simulink model "e5_3blocks_nn"  (R2020a)
settings: Solver=VariableStepAuto  StartTime=0.0  StopTime=10.0  RelTol=1e-3
undefined symbols (not defined in the file or in its folder): Quad
libraries: neural x123
(part 3 of 6)

== system e5_3blocks_nn/NN/Layer 2/Delays 1 ==
  "p{2}" : Inport  PortDimensions=50
      mask Display: e = 0.06;c1 = [120 230 180]/255;c2 = ([120 230 180]+0)/(256+128);c3 = ([120 230 180]+128)/(256+128);patch([0 1 1 0],[0 0 1 1],c1);patch([0 1 1 1-e 1-e 0+e],[0 0 1 1-e 0+e 0+e],c2);patch([0 0 1 1-e 0+e 0+e],[0 1 1 1-e 1-e 0+e],c3);plot([0 1 1 0 0],[0 0 1 1 0]);
  mux : Mux  Inputs=1
      mask Display: e = 0.06;c1 = [120 150 230]/255;c2 = ([120 150 230]+0)/383;c3 = ([120 150 230]+128)/383;patch([0 1 1 0],[0 0 1 1],c1);patch([0 1 1 1-e 1-e 0+e],[0 0 1 1-e 0+e 0+e],c2);patch([0 0 1 1-e 0+e 0+e],[0 1 1 1-e 1-e 0+e],c3);plot([0 1 1 0 0],[0 0 1 1 0]);disp('Mux')
  "pd{2,1}" : Outport
      mask Display: e = 0.06;c1 = [120 230 180]/255;c2 = ([120 230 180]+0)/(256+128);c3 = ([120 230 180]+128)/(256+128);patch([0 1 1 0],[0 0 1 1],c1);patch([0 1 1 1-e 1-e 0+e],[0 0 1 1-e 0+e 0+e],c2);patch([0 0 1 1-e 0+e 0+e],[0 1 1 1-e 1-e 0+e],c3);plot([0 1 1 0 0],[0 0 1 1 0]);
  wires:
  "p{2}"/1 -> mux/1
  mux/1 -> "pd{2,1}"/1

== system e5_3blocks_nn/NN/Layer 2/LW{2,1} ==
  "ad{2,1}" : Inport  PortDimensions=50
      mask Display: e = 0.06;c1 = [120 230 180]/255;c2 = ([120 230 180]+0)/(256+128);c3 = ([120 230 180]+128)/(256+128);patch([0 1 1 0],[0 0 1 1],c1);patch([0 1 1 1-e 1-e 0+e],[0 0 1 1-e 0+e 0+e],c2);patch([0 0 1 1-e 0+e 0+e],[0 1 1 1-e 1-e 0+e],c3);plot([0 1 1 0 0],[0 0 1 1 0]);
  "IW{2,1}(1,:)'" : Constant  Value=[0.06238826944898899495850486118797562085092067718505859375;-0.0662561883727814660005606128834187984466552734375;0.140596693924744442494301210899720899760723114013671875;0.3008382961340732020261157231288962066173553466796875;0.329270133314576940453122233520844019949436187744140625;-0.08899910732660483436706755355771747417747974395751953125;0.11667890650152978881948229172849096357822418212890625;-0.1929670553806901167614995529220323078334331512451171875;0.2111795311514239326111663785923155955970287322998046875;0.2287193471798081301216143401688896119594573974609375;-0.29845320395423546866453534676111303269863128662109375;-0.1754752706825663810530357977768289856612682342529296875;-0.234519474313424625133706058477400802075862884521484375;0.01548211534042116983844739053211014834232628345489501953125;-0.1728192200925544319556337313770200125873088836669921875;0.203750612111709583640362097867182455956935882568359375;-0.03263481715507744740367712665829458273947238922119140625;-0.0835109388646079475737593611484044231474399566650390625;-0.173454103671987935886278364705503918230533599853515625;-0.25354274639018326009676229659817181527614593505859375;0.05956454210532587112414404373339493758976459503173828125;-0.12377788023767373470906960619686287827789783477783203125;-0.048979806865181163555433840883779339492321014404296875;-0.0684319290588069339964505388707038946449756622314453125;0.2344023881326581515427420754349441267549991607666015625;0.0686577095032668005547549228140269406139850616455078125;0.0705147028712725665311467082574381493031978607177734375;0.311049450843584984749412569726700894534587860107421875;0.183230131462504053363460343462065793573856353759765625;0.081252526365822586029707963461987674236297607421875;-0.20765571332480303734513427116326056420803070068359375;0.02676877785194743675223350010128342546522617340087890625;0.30055041682881888931433422840200364589691162109375;0.09562847935589045833548738073659478686749935150146484375;0.1668647100894824486516654360457323491573333740234375;-0.0961144552936583351776533845622907392680644989013671875;-0.0312302350081472245013625155252157128416001796722412109375;-0.35432114836700978610650736300158314406871795654296875;0.1700429182737286104565299638124997727572917938232421875;-0.1468128720628165684303212401573546230792999267578125;0.32478039488932564093914834302267991006374359130859375;-0.2290287491159137822638314219148014672100543975830078125;-0.08672457421688405110327124702962464652955532073974609375;0.0266731992851400624700008989975685835815966129302978515625;0.1662091278922168957610239203859237022697925567626953125;0.2276717647203591876614581224202993325889110565185546875;0.199822119171683965088703871515463106334209442138671875;0.1305782909366972333042866694086114875972270965576171875;-0.0745158904154400725250440018498920835554599761962890625;-0.11266355005217280893514697481805342249572277069091796875]
      mask Display: e = 0.06;c1 = [120 150 230]/255;c2 = ([120 150 230]+0)/383;c3 = ([120 150 230]+128)/383;patch([0 1 1 0],[0 0 1 1],c1);patch([0 1 1 1-e 1-e 0+e],[0 0 1 1-e 0+e 0+e],c2);patch([0 0 1 1-e 0+e 0+e],[0 1 1 1-e 1-e 0+e],c3);plot([0 1 1 0 0],[0 0 1 1 0]);disp('weights');
  "IW{2,1}(2,:)'" : Constant  Value=[0.053859911191078267689302805365514359436929225921630859375;0.1116533205692238350792422352242283523082733154296875;-0.4240343441799243606737945810891687870025634765625;0.1368953708668934343695156030662474222481250762939453125;-0.0943260353503585780021722939636674709618091583251953125;0.171733416516677672714052960145636461675167083740234375;0.262014754263373450537955022809910587966442108154296875;0.04316320852678133535018645261516212485730648040771484375;-0.094505581266535354512114963654312305152416229248046875;0.1799789979013576568522836396368802525103092193603515625;-0.15630297243227875281235128568368963897228240966796875;0.12384955587173805680034632814567885361611843109130859375;0.1190447085715764241609093687657150439918041229248046875;0.263289083945134116948594282803242094814777374267578125;-0.1125910082716607141239961720202700234949588775634765625;-0.03594825728761497085628207059926353394985198974609375;-0.09538179906421283271722444396800710819661617279052734375;0.03382504542857060758631604358015465550124645233154296875;-0.09516068664822209532960783917587832547724246978759765625;-0.2472115131330177850710327902561402879655361175537109375;0.2200282479288944159634411334991455078125;-0.27077531053553050011117875328636728227138519287109375;0.11230775374953057277327417295964551158249378204345703125;0.10448450591650038088431529104127548635005950927734375;0.209030737108533870571847046448965556919574737548828125;-0.03888027185597515977821814203707617707550525665283203125;-0.2230029398786366190421404098742641508579254150390625;-0.2113154090177686850182681155274622142314910888671875;0.2253159625747749306157174942200072109699249267578125;-0.0759738296823943837221548847082885913550853729248046875;0.0232977391038076131479783725808374583721160888671875;0.0495270194348351455726486847197520546615123748779296875;-0.148411826106503053068763620103709399700164794921875;0.361210691757326285422635692157200537621974945068359375;-0.255217278371725975194550528613035567104816436767578125;-0.1139007461432639811693690035099280066788196563720703125;-0.131820962715450018531981868363800458610057830810546875;0.03699478200002949412894537317697540856897830963134765625;0.371812042058923708509610150940716266632080078125;0.238123332367356888017440041949157603085041046142578125;0.1813876888061571601706845058288308791816234588623046875;-0.04579007505833264379813130062757409177720546722412109375;-0.0142746944588547051979698920831651776097714900970458984375;-0.0505190325210966018065761318212025798857212066650390625;0.1416573248566437015494301476792315952479839324951171875;0.1885353697001486417139659579333965666592121124267578125;0.449669560775642296324150493092020042240619659423828125;0.07124427017188149358073445682748570106923580169677734375;0.0272623856827981791983717130278819240629673004150390625;-0.1683749712734463610530610822024755179882049560546875]
      mask Display: e = 0.06;c1 = [120 150 230]/255;c2 = ([120 150 230]+0)/383;c3 = ([120 150 230]+128)/383;patch([0 1 1 0],[0 0 1 1],c1);patch([0 1 1 1-e 1-e 0+e],[0 0 1 1-e 0+e 0+e],c2);patch([0 0 1 1-e 0+e 0+e],[0 1 1 1-e 1-e 0+e],c3);plot([0 1 1 0 0],[0 0 1 1 0]);disp('weights');
  Mux : Mux  Inputs=2
      mask Display: e = 0.06;c1 = [120 150 230]/255;c2 = ([120 150 230]+0)/383;c3 = ([120 150 230]+128)/383;patch([0 1 1 0],[0 0 1 1],c1);patch([0 1 1 1-e 1-e 0+e],[0 0 1 1-e 0+e 0+e],c2);patch([0 0 1 1-e 0+e 0+e],[0 1 1 1-e 1-e 0+e],c3);plot([0 1 1 0 0],[0 0 1 1 0]);disp('Mux');
  dotprod1 : neural/Weight Functions/dotprod
  dotprod2 : neural/Weight Functions/dotprod
  "lz{2,1}" : Outport
      mask Display: e = 0.06;c1 = [120 230 180]/255;c2 = ([120 230 180]+0)/(256+128);c3 = ([120 230 180]+128)/(256+128);patch([0 1 1 0],[0 0 1 1],c1);patch([0 1 1 1-e 1-e 0+e],[0 0 1 1-e 0+e 0+e],c2);patch([0 0 1 1-e 0+e 0+e],[0 1 1 1-e 1-e 0+e],c3);plot([0 1 1 0 0],[0 0 1 1 0]);
  wires:
  "IW{2,1}(1,:)'"/1 -> dotprod1/1
  "ad{2,1}"/1 -> dotprod1/2, dotprod2/2
  dotprod1/1 -> Mux/1
  "IW{2,1}(2,:)'"/1 -> dotprod2/1
  dotprod2/1 -> Mux/2
  Mux/1 -> "lz{2,1}"/1

== system e5_3blocks_nn/NN_online/Layer 1/Delays 1 ==
  "p{1}" : Inport  PortDimensions=20
      mask Display: e = 0.06;c1 = [120 230 180]/255;c2 = ([120 230 180]+0)/(256+128);c3 = ([120 230 180]+128)/(256+128);patch([0 1 1 0],[0 0 1 1],c1);patch([0 1 1 1-e 1-e 0+e],[0 0 1 1-e 0+e 0+e],c2);patch([0 0 1 1-e 0+e 0+e],[0 1 1 1-e 1-e 0+e],c3);plot([0 1 1 0 0],[0 0 1 1 0]);
  mux : Mux  Inputs=1
      mask Display: e = 0.06;c1 = [120 150 230]/255;c2 = ([120 150 230]+0)/383;c3 = ([120 150 230]+128)/383;patch([0 1 1 0],[0 0 1 1],c1);patch([0 1 1 1-e 1-e 0+e],[0 0 1 1-e 0+e 0+e],c2);patch([0 0 1 1-e 0+e 0+e],[0 1 1 1-e 1-e 0+e],c3);plot([0 1 1 0 0],[0 0 1 1 0]);disp('Mux')
  "pd{1,1}" : Outport
      mask Display: e = 0.06;c1 = [120 230 180]/255;c2 = ([120 230 180]+0)/(256+128);c3 = ([120 230 180]+128)/(256+128);patch([0 1 1 0],[0 0 1 1],c1);patch([0 1 1 1-e 1-e 0+e],[0 0 1 1-e 0+e 0+e],c2);patch([0 0 1 1-e 0+e 0+e],[0 1 1 1-e 1-e 0+e],c3);plot([0 1 1 0 0],[0 0 1 1 0]);
  wires:
  "p{1}"/1 -> mux/1
  mux/1 -> "pd{1,1}"/1
